simulink model "E_InputWaterFlowControl"  (R2017a)
settings: Solver=VariableStepAuto  StartTime=0.0  StopTime=30  MaxStep=1e-3  RelTol=1e-3  EnableMultiTasking=on
InitFcn:
  | S1=20;
  | S2=20;
  | h1=5;
  | h2=5;
  | A=31;
  | B=25;
libraries: fuzblock x1
settings Model: Creator=Hossein  LastModifiedBy=h.zolfaghari
settings OptimizationCC: LifeSpan=inf
settings DebuggingCC: SFUnexpectedBacktrackingDiag=warning  SFNoUnconditionalDefaultTransitionDiag=warning  SFExecutionAtInitializationDiag=none
settings GRTTargetCC: TargetLangStandard=C89/C90 (ANSI)  GeneratePreprocessorConditionals=Disable all
settings ConfigComp: CovMetricSettings=dw  CovHtmlReporting=on  CovSaveCumulativeToWorkspaceVar=on  CovSaveSingleToWorkspaceVar=on  CovExternalEMLEnable=off

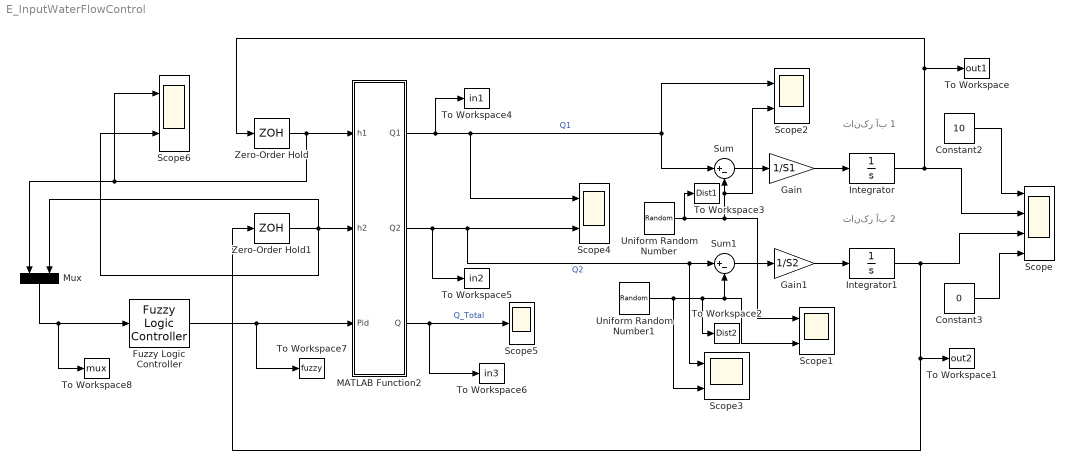
== system E_InputWaterFlowControl ==
  note: تانکر آب 1
  note: تانکر آب 2
  Constant2 : Constant  Value=10
  Constant3 : Constant  Value=0
  Fuzzy Logic Controller : fuzblock/Fuzzy Logic  Controller  fis=NFIS
  Gain : Gain  Gain=1/S1
  Gain1 : Gain  Gain=1/S2
  Integrator : Integrator  InitialCondition=h1
  Integrator1 : Integrator  InitialCondition=h2
  MATLAB Function2 : MATLAB Function  TreatAsAtomicUnit=on
  Mux : Mux  Inputs=2
  Scope : Scope  NumInputPorts=4
  Scope{1..4,6} (5 alike) : Scope  NumInputPorts=2
  Scope5 : Scope
  Sum : Sum  Inputs=|+-
  Sum1 : Sum  Inputs=|+-
  To Workspace : ToWorkspace  VariableName=out1  SaveFormat=Timeseries  SampleTime=-1
  To Workspace1 : ToWorkspace  VariableName=out2  SaveFormat=Timeseries  SampleTime=-1
  To Workspace2 : ToWorkspace  VariableName=Dist2  SaveFormat=Timeseries  SampleTime=-1
  To Workspace3 : ToWorkspace  VariableName=Dist1  SaveFormat=Timeseries  SampleTime=-1
  To Workspace4 : ToWorkspace  VariableName=in1  SaveFormat=Timeseries  SampleTime=-1
  To Workspace5 : ToWorkspace  VariableName=in2  SaveFormat=Timeseries  SampleTime=-1
  To Workspace6 : ToWorkspace  VariableName=in3  SaveFormat=Timeseries  SampleTime=-1
  To Workspace7 : ToWorkspace  VariableName=fuzzy  SaveFormat=Timeseries  SampleTime=-1
  To Workspace8 : ToWorkspace  VariableName=mux  SaveFormat=Timeseries  SampleTime=-1
  Uniform Random Number : UniformRandomNumber  Minimum=A*0.9  Maximum=A*1.1  Seed=randi([1,5])  SampleTime=1
  Uniform Random Number1 : UniformRandomNumber  Minimum=B*0.9  Maximum=B*1.1  Seed=randi([1,5])  SampleTime=0.3
  Zero-Order Hold : ZeroOrderHold  SampleTime=0.01
  Zero-Order Hold1 : ZeroOrderHold  SampleTime=0.01
  wires:
  MATLAB Function2/1(Q1) -> To Workspace4/1, Scope4/1, Sum/1, Scope2/1  "Q1"
  MATLAB Function2/2(Q2) -> To Workspace5/1, Scope3/1, Sum1/1, Scope4/2  "Q2"
  Sum/1 -> Gain/1
  Gain/1 -> Integrator/1
  Gain1/1 -> Integrator1/1
  Sum1/1 -> Gain1/1
  Integrator/1 -> To Workspace/1, Zero-Order Hold/1, Scope/2
  Integrator1/1 -> To Workspace1/1, Zero-Order Hold1/1, Scope/3
  Constant2/1 -> Scope/1
  Constant3/1 -> Scope/4
  Uniform Random Number/1 -> To Workspace3/1, Scope1/1, Scope2/2, Sum/2
  Uniform Random Number1/1 -> Scope3/2, To Workspace2/1, Scope1/2, Sum1/2
  Zero-Order Hold/1 -> Mux/1, Scope6/1, MATLAB Function2/1(h1)
  Zero-Order Hold1/1 -> Mux/2, Scope6/2, MATLAB Function2/2(h2)
  MATLAB Function2/3(Q) -> To Workspace6/1, Scope5/1  "Q_Total"
  Fuzzy Logic Controller/1 -> To Workspace7/1, MATLAB Function2/3(Pid)
  Mux/1 -> To Workspace8/1, Fuzzy Logic Controller/1

== matlab function E_InputWaterFlowControl/MATLAB Function2 ==
  data: h1 input; Q1 output; Q2 output; h2 input; Pid input; Q output
function [Q1,Q2,Q] = fcn(h1,h2, Pid)
%#codegen
    % Q is Q1
     persistent q1 


     if isempty(q1)
         q1=25; 
     end
    
 Q1=q1;
    if h1>h2
        Q1=Q1*0.996;
    else
        Q1=Q1*1.004;
    end
 q1=Q1;
 Q=50*Pid;
 
 if Q>=60
     Q=60;
 end
 Q2=Q-q1;
